simulink model "EJEMPLO_MATLAB"  (R2017b)
settings: Solver=FixedStepAuto  StartTime=0.0  StopTime=inf  RelTol=1e-3
libraries: instrumentlib x1
settings Model: Creator=Juan Ricardo  LastModifiedBy=Juan Ricardo

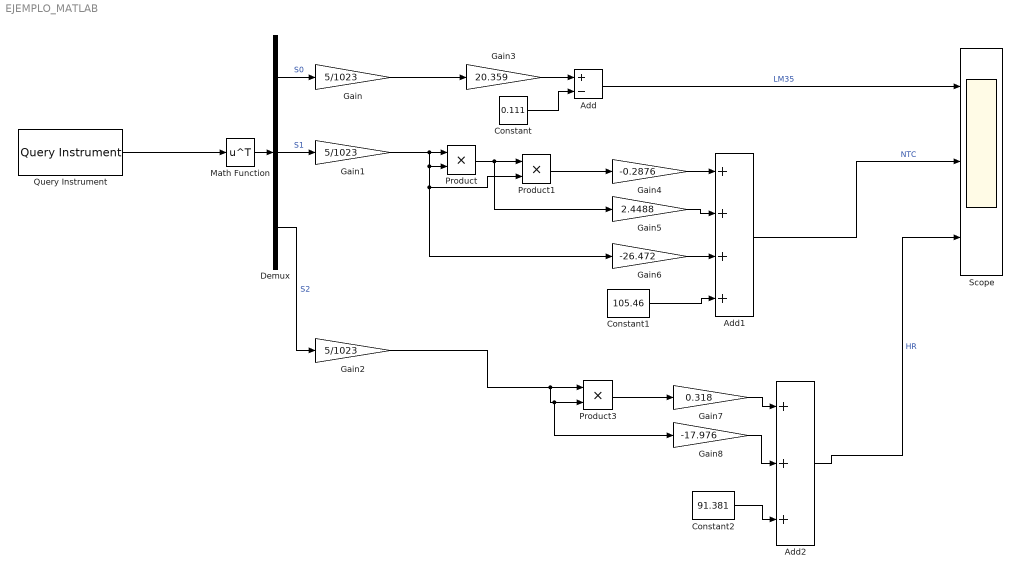
== system EJEMPLO_MATLAB ==
  Add : Sum  Inputs=+-
  Add1 : Sum  Inputs=++++
  Add2 : Sum  Inputs=+++
  Constant : Constant  Value=0.111
  Constant1 : Constant  Value=105.46
  Constant2 : Constant  Value=91.381
  Demux : Demux  Outputs=3
  Gain : Gain  Gain=5/1023
  Gain1 : Gain  Gain=5/1023
  Gain2 : Gain  Gain=5/1023
  Gain3 : Gain  Gain=20.359
  Gain4 : Gain  Gain=-0.2876
  Gain5 : Gain  Gain=2.4488
  Gain6 : Gain  Gain=-26.472
  Gain7 : Gain  Gain=0.318
  Gain8 : Gain  Gain=-17.976
  Math Function : Math  Operator=transpose  SaturateOnIntegerOverflow=on
  Product : Product
  Product1 : Product
  Product3 : Product
  Query Instrument : instrumentlib/Query Instrument  sampleTime=0.04992  isWorkspaceObject=off  timeout=10  inputBufferSize=8192  protocol=Serial  serialPort=COM2  baudRate=9600  gpibVendor=Agilent Technologies  boardIndex=0  primaryAddress=1  secondaryAddress=0  visaVendor=Agilent  visaSerialPort=0  chassisIndex=0  logicalAddress=0  tcpRemoteHost='127.0.0.1'  tcpRemotePort=4500  udpRemoteHost='127.0.0.1'  udpRemotePort=9090  visaTCPBoardIndex=0  visaTCPRemoteHost='127.0.0.1'  usbBoardIndex=0  usbManufID=0  usbModelCode=0  usbSerialNumber=0  initAction=None  initCommand='DATA:SOURCE CH1'  initFunction=get  queryCommand=''  responseFormat=ASCII  asciiFormatting='S%d,%d,%d'  precision=8-bit integer  byteOrder=Little endian  valuesToRead=1  removeBytes=off  afterOutputAction=Repeat query for new data  enableFrames=on  frameSize=3
      settings: SourceProductName=Instrument Control Toolbox  SourceProductBaseCode=IC
  Scope : Scope  NumInputPorts=3
  wires:
  Query Instrument/1 -> Math Function/1
  Math Function/1 -> Demux/1
  Demux/1 -> Gain/1  "S0"
  Demux/2 -> Gain1/1  "S1"
  Demux/3 -> Gain2/1  "S2"
  Gain/1 -> Gain3/1
  Gain3/1 -> Add/1
  Constant/1 -> Add/2
  Add/1 -> Scope/1  "LM35"
  Product/1 -> Gain5/1, Product1/1
  Gain1/1 -> Gain6/1, Product1/2, Product/2, Product/1
  Product1/1 -> Gain4/1
  Gain4/1 -> Add1/1
  Gain5/1 -> Add1/2
  Gain6/1 -> Add1/3
  Constant1/1 -> Add1/4
  Add1/1 -> Scope/2  "NTC"
  Product3/1 -> Gain7/1
  Gain7/1 -> Add2/1
  Constant2/1 -> Add2/3
  Gain8/1 -> Add2/2
  Gain2/1 -> Gain8/1, Product3/2, Product3/1
  Add2/1 -> Scope/3  "HR"
